simulink model "Neurofeedback_ErrorFunction_ConnectivityChanges"  (R2021b)
settings: Solver=VariableStepAuto  StartTime=0.0  StopTime=30  RelTol=1e-3
settings Model: Creator=mariodelossantos  LastModifiedBy=mariodelossantos

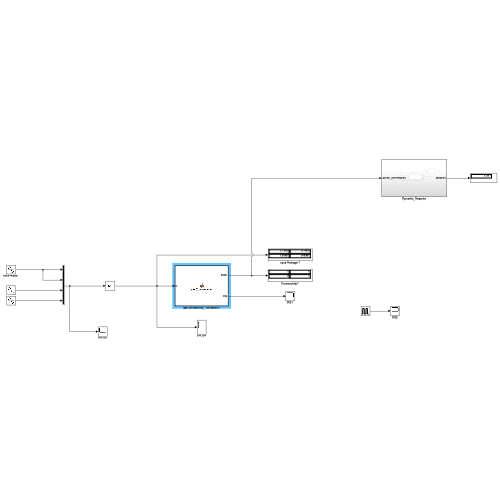
[thumbnail: Simulink's stored preview of the top-level diagram]
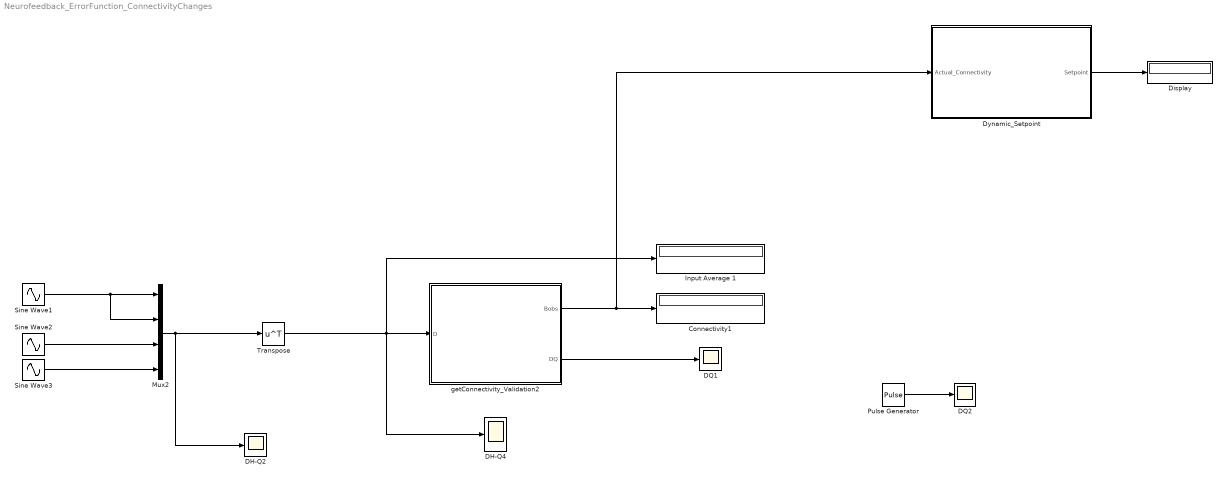
== system Neurofeedback_ErrorFunction_ConnectivityChanges ==
  Connectivity1 : Display
  DH-Q2 : Scope
  DH-Q4 : Scope
  DQ1 : Scope
  DQ2 : Scope
  Display : Display
  Dynamic_Setpoint : Subsystem
  Input Average 1 : Display
  Mux2 : Mux
  Pulse Generator : DiscretePulseGenerator  PulseType=Time based  Period=10  PulseWidth=5
  Sine Wave1 : Sin  Amplitude=1.2  SampleTime=0
  Sine Wave2 : Sin  Frequency=1.4  SampleTime=0
  Sine Wave3 : Sin  Frequency=1.4  SampleTime=0
  Transpose : Math  Operator=transpose  SaturateOnIntegerOverflow=on
  getConnectivity_Validation2 : MATLAB Function  TreatAsAtomicUnit=on  SystemSampleTime=0
  wires:
  Mux2/1 -> DH-Q2/1, Transpose/1
  Transpose/1 -> DH-Q4/1, getConnectivity_Validation2/1("D "), Input Average 1/1
  getConnectivity_Validation2/2(DQ) -> DQ1/1
  getConnectivity_Validation2/1(Bobs) -> Dynamic_Setpoint/1(Actual_Connectivity), Connectivity1/1
  Sine Wave2/1 -> Mux2/3
  Sine Wave3/1 -> Mux2/4
  Sine Wave1/1 -> Mux2/2, Mux2/1
  Pulse Generator/1 -> DQ2/1
  Dynamic_Setpoint/1(Setpoint) -> Display/1

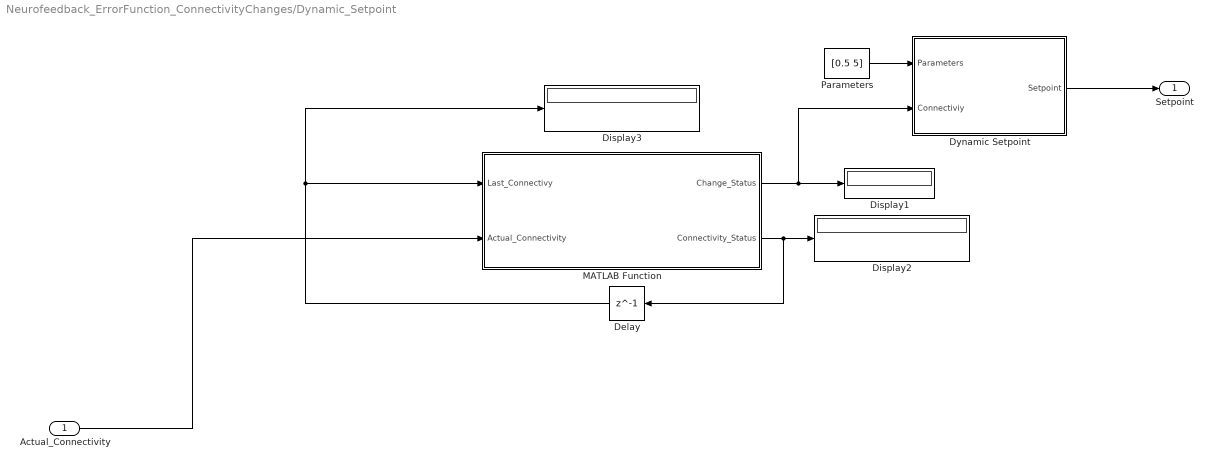
== system Neurofeedback_ErrorFunction_ConnectivityChanges/Dynamic_Setpoint ==
  Actual_Connectivity : Inport
  Delay : Delay  DelayLength=1
  Display1 : Display
  Display2 : Display
  Display3 : Display
  Dynamic Setpoint : Subsystem
  MATLAB Function : MATLAB Function  TreatAsAtomicUnit=on
  Parameters : Constant  Value=[0.5 5]
  Setpoint : Outport
  wires:
  Dynamic Setpoint/1(Setpoint) -> Setpoint/1
  Actual_Connectivity/1 -> MATLAB Function/2(Actual_Connectivity)
  MATLAB Function/2(Connectivity_Status) -> Display2/1, Delay/1
  Delay/1 -> Display3/1, MATLAB Function/1(Last_Connectivy)
  Parameters/1 -> Dynamic Setpoint/1(Parameters)
  MATLAB Function/1(Change_Status) -> Dynamic Setpoint/2(Connectiviy), Display1/1

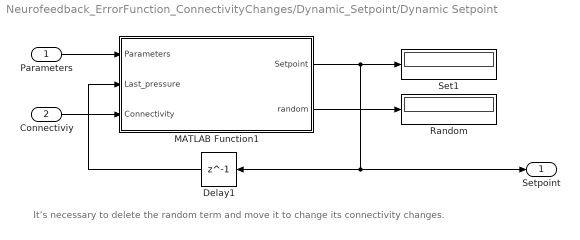
== system Neurofeedback_ErrorFunction_ConnectivityChanges/Dynamic_Setpoint/Dynamic Setpoint ==
  note: It’s necessary to delete the random term and move it to change its connectivity changes.
  Parameters : Inport
  Connectiviy : Inport  Port=2
  Delay1 : Delay  DelayLength=1  InitialCondition=0
  MATLAB Function1 : MATLAB Function  TreatAsAtomicUnit=on
  Random : Display
  Set1 : Display
  Setpoint : Outport
  wires:
  Parameters/1 -> MATLAB Function1/1(Parameters)
  MATLAB Function1/2(random) -> Random/1
  MATLAB Function1/1(Setpoint) -> Set1/1, Setpoint/1, Delay1/1
  Delay1/1 -> MATLAB Function1/2(Last_pressure)
  Connectiviy/1 -> MATLAB Function1/3(Connectivity)

== matlab function Neurofeedback_ErrorFunction_ConnectivityChanges/Dynamic_Setpoint/MATLAB Function ==
  data: Last_Connectivy input boolean; Change_Status output; Actual_Connectivity input; Connectivity_Status output
function [Change_Status, Connectivity_Status] = Connectivity_Changes(Last_Connectivy , Actual_Connectivity)

if(Actual_Connectivity == Last_Connectivy)
    Change_Status = 0;
    
else
    Change_Status = 1;
end

Connectivity_Status = Actual_Connectivity;

== matlab function Neurofeedback_ErrorFunction_ConnectivityChanges/getConnectivity_Validation2 ==
  data: D input; Bobs output; DQ output
function [Bobs,DQ]  = getConnectivity(D)

    DQ = zeros(1, 2);
    DQ(1,1)=D(1,1);
    DQ(1,2)=D(1,2);


    DH = zeros(1,2);
    DH(1,1)=D(1,3);
    DH(1,2)=D(1,4);

    rThresh= 0.6; % [0..1] A threshold on the correlation.

    [nSamples, nChannels, nHb]=size(DQ);

    C = nan(nChannels, nChannels, nHb); %Matrix of channel pairwise correlations;

    %This part of the algorithm is HIGHLY inefficient but it does the job for now
    %but might not be sufficiently fast for "real time" neurofeedback

    for iHb = 1:nHb
        for iCh=1:nChannels
            for jCh=iCh:nChannels

                if iCh == jCh

                 C(iCh,jCh,iHb) = 1;

               else

                 C(iCh,jCh,iHb) = xcorr2(DQ(:,iCh,iHb),DQ(:,jCh,iHb));

                end
            end

        end

    end

    %Threshold/Binarize C


    tmp = C > rThresh;

    %Finally "merge" accross Hb species

    Bobs = all(tmp,3); %Apply the AND function across Hb species.

== matlab function Neurofeedback_ErrorFunction_ConnectivityChanges/Dynamic_Setpoint/Dynamic Setpoint/MATLAB Function1 ==
  settings: updateMethod=DISCRETE
  data: Setpoint output; Parameters input; Last_pressure input; random output; Connectivity input
function [Setpoint, random] = Random_Setpoint(Parameters, Last_pressure, Connectivity)
    %Parameters = [threshold Start_setpoint]
    temp = 0;
   %Pressure Setpoint selection
    pmin = 5;
    pmax = 8;
    new_pressure = pmin + rand(1)*(pmax-pmin);

    %Random used to simulate the connectivity changes, so we must change
    %the pressure setpoint when changes in the connectitvy are observed.
    min = 0;
    tmax = 10;
        %We should fine a random criteria to change the setpoint, not just
        %time, or the moment B changes. For now works to demostrate the
        %control without fNIRS
    random = min + rand(1) * (tmax - min) * new_pressure;
    if (Connectivity == 1)
         %if (random < Parameters(1))
            %disp("Time")
            %disp(Time)
            temp = new_pressure;
            %disp("Setpoint")
            %disp(temp)
        %else 
            %temp = Last_pressure;
%                 if (Parameters(2) == temp || temp == 0)
%                     temp = Parameters(2);
%                 else
%                     temp = Last_pressure;
%                 end
    else
        temp = Last_pressure;
    end

    Setpoint = temp;
